simulink model "twoP"  (R2016b)
settings: Solver=FixedStepAuto  StartTime=0.0  StopTime=simstop  MaxStep=0.1  RelTol=1e-3  EnableMultiTasking=on
values from neighbouring files (symbols this model uses):
  CV01 = 100    [PIDValveTest.m]    (also in PIDtestP2m.m; loggingTest.m)
  simstop = 60*1    (= 60)    [PIDValveTest.m]    (also in PIDtestP2m.m; gatherData.m = WPtime(end)+(WPtime(end)-WPtime(end-1)))
libraries: slrtlib x5, xpcnilib x2, powerlib_meascontrol x1
settings Model: ModifiedByFormat=The MathWorks Inc.  Creator=The MathWorks, Inc.  LastModifiedBy=The MathWorks Inc.
settings SolverCC: EnableConcurrentExecution=on
settings DataIOCC: LimitDataPoints=on  SaveFormat=Array
settings OptimizationCC: BlockReduction=off  DefaultParameterBehavior=Inlined  OptimizeBlockIOStorage=off  BufferReuse=off  GlobalBufferReuse=off  ExpressionFolding=off  ExpressionDepthLimit=2147483647  LocalBlockOutputs=off  LifeSpan=inf
settings DebuggingCC: UnderspecifiedInitializationDetection=Classic  MergeDetectMultiDrivingBlocksExec=none  SolverPrmCheckMsg=warning  FcnCallInpInsideContextMsg=warning  AllowSymbolicDim=off  StateNameClashWarn=warning  SFUnexpectedBacktrackingDiag=warning  SFNoUnconditionalDefaultTransitionDiag=warning  SFExecutionAtInitializationDiag=none
settings HardwareCC: ProdBitPerPointer=32  ProdBitPerSizeT=32  ProdBitPerPtrDiffT=32  ProdLargestAtomicFloat=None  ProdWordSize=32  ProdLongLongMode=on  ProdHWDeviceType=Generic->32-bit x86 compatible
settings ModelReferenceCC: ModelReferenceNumInstancesAllowed=Single  ModelReferenceMinAlgLoopOccurrences=on  PropagateSignalLabelsOutOfModel=off
settings RTWCC: SystemTargetFile=slrt.tlc  TemplateMakefile=slrt_default_tmf  Description=Simulink Real-Time  RTWVerbose=off
settings ConfigComp: CovMetricSettings=dw  CovHtmlReporting=on  CovSaveCumulativeToWorkspaceVar=on  CovSaveSingleToWorkspaceVar=on  CovExternalEMLEnable=off  CovSFcnEnable=off

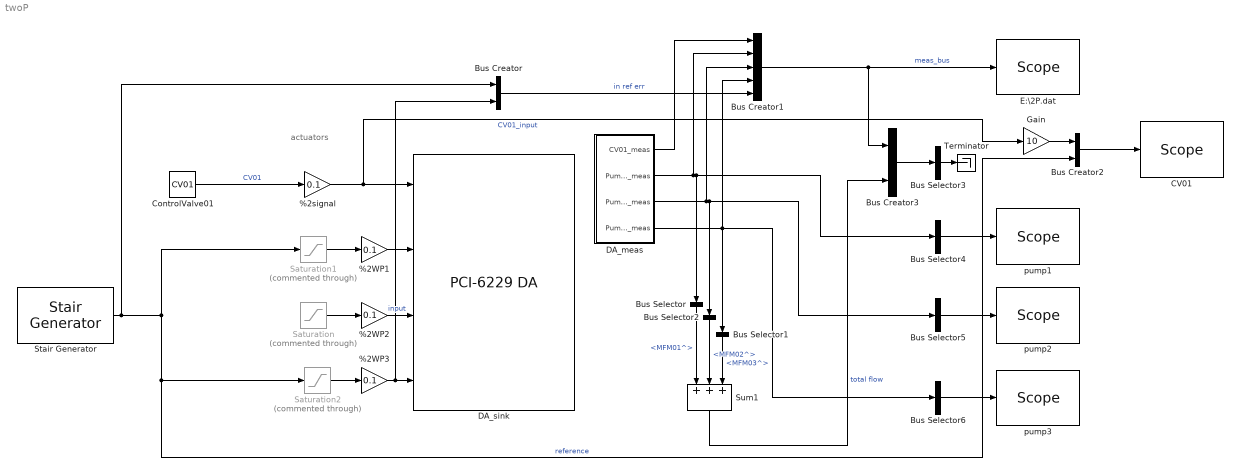
== system twoP ==
  note: actuators
  %2WP1 : Gain  Gain=0.1
  %2WP2 : Gain  Gain=0.1
  %2WP3 : Gain  Gain=0.1
  %2signal : Gain  Gain=0.1
  Bus Creator : BusCreator  Inputs=2
  Bus Creator1 : BusCreator  Inputs=5
  Bus Creator2 : BusCreator  Inputs=2
  Bus Creator3 : BusCreator  Inputs=2
  Bus Selector : BusSelector  OutputSignals=MFM01^
  Bus Selector1 : BusSelector  OutputSignals=MFM03^
  Bus Selector2 : BusSelector  OutputSignals=MFM02^
  Bus Selector3 : BusSelector  OutputSignals=meas_bus.Pump1.MFM01^  OutputAsBus=on
  Bus Selector4 : BusSelector  OutputSignals=DPT01,MFM01^  OutputAsBus=on
  Bus Selector5 : BusSelector  OutputSignals=DPT02,MFM02^  OutputAsBus=on
  Bus Selector6 : BusSelector  OutputSignals=DPT03,MFM03^  OutputAsBus=on
  CV01 : slrtlib/Displays and Logging/Scope   scopeno=4  scopetype=Target  autostart=on  viewmode=Graphical sliding  formatstr='%1.0g'  grid=on  ylimits=[0,100]  nosamples=100*simstop  noprepostsamples=0  interleave=1  triggermode=FreeRun  triggersignal=1  trigsignalfromport=on  triggerlevel=0.0  triggerslope=Either  triggerscope=1  triggersample=0  filename=E:\unused1.dat  mode=Lazy  writesize=512  autorestart=off  dynamicfilemode=off  maxwritefilesize=512*1024^2
  ControlValve01 : Constant  Value=CV01
  DA_meas : Subsystem
  DA_sink : xpcnilib/D//A/M Series/PCI-6229 DA  channel=[4 1 2 3]  reset=[1]  initValue=[0]  sampletime=0.01  slot=-1
  E:\2P.dat : slrtlib/Displays and Logging/Scope   scopeno=20  scopetype=File  autostart=on  viewmode=Graphical sliding  formatstr='%15.6f'  grid=on  ylimits=[0,0]  nosamples=100*simstop  noprepostsamples=0  interleave=1  triggermode=FreeRun  triggersignal=1  trigsignalfromport=off  triggerlevel=0.0  triggerslope=Either  triggerscope=1  triggersample=0  filename=E:\2P.dat  mode=Commit  writesize=512  autorestart=off  dynamicfilemode=off  maxwritefilesize=512*1024^2
  Gain : Gain  Gain=10
  Saturation : Saturate  Commented=through  UpperLimit=80  LowerLimit=0
  Saturation1 : Saturate  Commented=through  UpperLimit=80  LowerLimit=0
  Saturation2 : Saturate  Commented=through  UpperLimit=80  LowerLimit=0
  Stair Generator : powerlib_meascontrol/Pulse & Signal Generators/Stair Generator  t=WPtime  e=WP2  Ts=0
  Sum1 : Sum  Inputs=+++
  Terminator : Terminator
  pump1 : slrtlib/Displays and Logging/Scope   scopeno=1  scopetype=Target  autostart=on  viewmode=Graphical sliding  formatstr='%15.6f'  grid=on  ylimits=[0,0]  nosamples=100*simstop  noprepostsamples=0  interleave=1  triggermode=FreeRun  triggersignal=1  trigsignalfromport=off  triggerlevel=0.0  triggerslope=Either  triggerscope=1  triggersample=0  filename=E:\unused1.dat  mode=Lazy  writesize=512  autorestart=off  dynamicfilemode=off  maxwritefilesize=512*1024^2
  pump2 : slrtlib/Displays and Logging/Scope   scopeno=2  scopetype=Target  autostart=on  viewmode=Graphical sliding  formatstr='%15.6f'  grid=on  ylimits=[0,0]  nosamples=100*simstop  noprepostsamples=0  interleave=1  triggermode=FreeRun  triggersignal=1  trigsignalfromport=off  triggerlevel=0.0  triggerslope=Either  triggerscope=1  triggersample=0  filename=E:\unused1.dat  mode=Lazy  writesize=512  autorestart=off  dynamicfilemode=off  maxwritefilesize=512*1024^2
  pump3 : slrtlib/Displays and Logging/Scope   scopeno=3  scopetype=Target  autostart=on  viewmode=Graphical sliding  formatstr='%15.6f'  grid=on  ylimits=[0,0]  nosamples=100*simstop  noprepostsamples=0  interleave=1  triggermode=FreeRun  triggersignal=1  trigsignalfromport=off  triggerlevel=0.0  triggerslope=Either  triggerscope=1  triggersample=0  filename=E:\unused1.dat  mode=Lazy  writesize=512  autorestart=off  dynamicfilemode=off  maxwritefilesize=512*1024^2
  wires:
  %2signal/1 -> Gain/1, DA_sink/1  "CV01_input"
  %2WP1/1 -> DA_sink/2
  %2WP3/1 -> Bus Creator/2, DA_sink/4
  DA_meas/4(Pump3_meas) -> Bus Selector6/1, Bus Creator1/4, Bus Selector1/1
  DA_meas/2(Pump1_meas) -> Bus Selector4/1, Bus Selector/1, Bus Creator1/2
  DA_meas/3(Pump2_meas) -> Bus Selector5/1, Bus Selector2/1, Bus Creator1/3
  Bus Creator1/1 -> Bus Creator3/1, E:\2P.dat/1  "meas_bus"
  Bus Selector/1 -> Sum1/1  "<MFM01^>"
  Bus Selector2/1 -> Sum1/2  "<MFM02^>"
  Bus Selector1/1 -> Sum1/3  "<MFM03^>"
  Sum1/1 -> Bus Creator3/2  "total flow"
  %2WP2/1 -> DA_sink/3  "input"
  Stair Generator/1 -> Saturation1/1, Saturation2/1, Bus Creator2/2, Bus Creator/1  "reference"
  Saturation/1 -> %2WP2/1
  Bus Creator3/1 -> Bus Selector3/1
  DA_meas/1(CV01_meas) -> Bus Creator1/1
  Bus Creator/1 -> Bus Creator1/5  "in ref err"
  Saturation1/1 -> %2WP1/1
  Saturation2/1 -> %2WP3/1
  ControlValve01/1 -> %2signal/1  "CV01"
  Bus Selector4/1 -> pump1/1
  Bus Selector5/1 -> pump2/1
  Bus Selector6/1 -> pump3/1
  Bus Creator2/1 -> CV01/1
  Bus Selector3/1 -> Terminator/1
  Gain/1 -> Bus Creator2/1

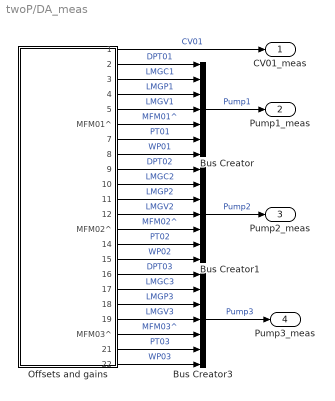
== system twoP/DA_meas ==
  Bus Creator : BusCreator  Inputs=7
  Bus Creator1 : BusCreator  Inputs=7
  Bus Creator3 : BusCreator  Inputs=7
  Offsets and gains : Subsystem
  CV01_meas : Outport
  Pump1_meas : Outport  Port=2
  Pump2_meas : Outport  Port=3
  Pump3_meas : Outport  Port=4
  wires:
  Bus Creator/1 -> Pump1_meas/1  "Pump1"
  Bus Creator1/1 -> Pump2_meas/1  "Pump2"
  Bus Creator3/1 -> Pump3_meas/1  "Pump3"
  Offsets and gains/8(8) -> Bus Creator/7  "WP01"
  Offsets and gains/9(9) -> Bus Creator1/1  "DPT02"
  Offsets and gains/4(4) -> Bus Creator/3  "LMGP1"
  Offsets and gains/2(2) -> Bus Creator/1  "DPT01"
  Offsets and gains/1(1) -> CV01_meas/1  "CV01"
  Offsets and gains/11(11) -> Bus Creator1/3  "LMGP2"
  Offsets and gains/15(15) -> Bus Creator1/7  "WP02"
  Offsets and gains/18(18) -> Bus Creator3/3  "LMGP3"
  Offsets and gains/22(22) -> Bus Creator3/7  "WP03"
  Offsets and gains/6(MFM01^) -> Bus Creator/5  "MFM01^"
  Offsets and gains/20(MFM03^) -> Bus Creator3/5  "MFM03^"
  Offsets and gains/10(10) -> Bus Creator1/2  "LMGC2"
  Offsets and gains/12(12) -> Bus Creator1/4  "LMGV2"
  Offsets and gains/13(MFM02^) -> Bus Creator1/5  "MFM02^"
  Offsets and gains/14(14) -> Bus Creator1/6  "PT02"
  Offsets and gains/19(19) -> Bus Creator3/4  "LMGV3"
  Offsets and gains/21(21) -> Bus Creator3/6  "PT03"
  Offsets and gains/16(16) -> Bus Creator3/1  "DPT03"
  Offsets and gains/17(17) -> Bus Creator3/2  "LMGC3"
  Offsets and gains/3(3) -> Bus Creator/2  "LMGC1"
  Offsets and gains/5(5) -> Bus Creator/4  "LMGV1"
  Offsets and gains/7(7) -> Bus Creator/6  "PT01"

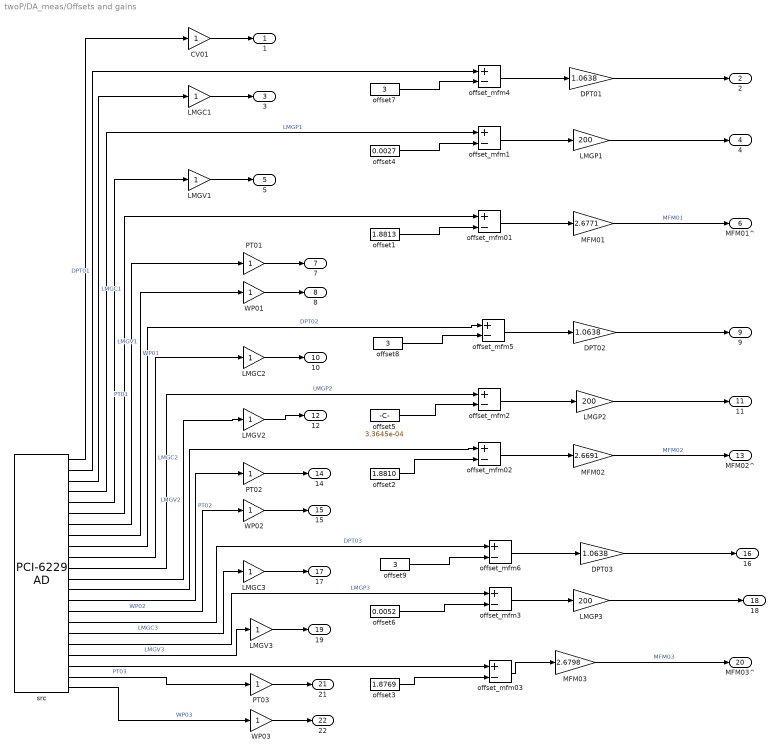
== system twoP/DA_meas/Offsets and gains ==
  CV01 : Gain
  DPT01 : Gain  Gain=1.0638
  DPT02 : Gain  Gain=1.0638
  DPT03 : Gain  Gain=1.0638
  LMGC1 : Gain
  LMGC2 : Gain
  LMGC3 : Gain
  LMGP1 : Gain  Gain=200
  LMGP2 : Gain  Gain=200
  LMGP3 : Gain  Gain=200
  LMGV1 : Gain
  LMGV2 : Gain
  LMGV3 : Gain
  MFM01 : Gain  Gain=2.6771
  MFM02 : Gain  Gain=2.6691
  MFM03 : Gain  Gain=2.6798
  PT01 : Gain
  PT02 : Gain
  PT03 : Gain
  WP01 : Gain
  WP02 : Gain
  WP03 : Gain
  offset1 : Constant  Value=1.8813
  offset2 : Constant  Value=1.8810
  offset3 : Constant  Value=1.8769
  offset4 : Constant  Value=0.0027
  offset5 : Constant  Value=3.3645e-04
  offset6 : Constant  Value=0.0052
  offset7 : Constant  Value=3
  offset8 : Constant  Value=3
  offset9 : Constant  Value=3
  offset_mfm01 : Sum  Inputs=+-
  offset_mfm02 : Sum  Inputs=+-
  offset_mfm03 : Sum  Inputs=+-
  offset_mfm{1..6} (6 alike) : Sum  Inputs=+-
  src : xpcnilib/A//D/M Series/PCI-6229 AD  channel=[4 17 5 11 8 21 24 1 18 6 12 9 22 25 2 19 7 13 10 23 26 3]  range=[10]  coupling=[0]  scantime=5e-6  sampletime=0.01  slot=-1
  1 : Outport
  2 : Outport  Port=2
  3 : Outport  Port=3
  4 : Outport  Port=4
  5 : Outport  Port=5
  MFM01^ : Outport  Port=6
  7 : Outport  Port=7
  8 : Outport  Port=8
  9 : Outport  Port=9
  10 : Outport  Port=10
  11 : Outport  Port=11
  12 : Outport  Port=12
  MFM02^ : Outport  Port=13
  14 : Outport  Port=14
  15 : Outport  Port=15
  16 : Outport  Port=16
  17 : Outport  Port=17
  18 : Outport  Port=18
  19 : Outport  Port=19
  MFM03^ : Outport  Port=20
  21 : Outport  Port=21
  22 : Outport  Port=22
  wires:
  src/18 -> offset_mfm3/1  "LMGP3"
  src/19 -> LMGV3/1  "LMGV3"
  src/22 -> WP03/1  "WP03"
  src/21 -> PT03/1  "PT03"
  src/10 -> LMGC2/1  "LMGC2"
  src/12 -> LMGV2/1  "LMGV2"
  src/15 -> WP02/1  "WP02"
  src/3 -> LMGC1/1  "LMGC1"
  src/9 -> offset_mfm5/1  "DPT02"
  src/11 -> offset_mfm2/1  "LMGP2"
  src/14 -> PT02/1  "PT02"
  src/16 -> offset_mfm6/1  "DPT03"
  src/17 -> LMGC3/1  "LMGC3"
  src/2 -> offset_mfm4/1  "DPT01"
  src/1 -> CV01/1
  MFM03/1 -> MFM03^/1  "MFM03"
  offset1/1 -> offset_mfm01/2
  src/4 -> offset_mfm1/1  "LMGP1"
  src/5 -> LMGV1/1  "LMGV1"
  src/7 -> PT01/1  "PT01"
  src/8 -> WP01/1  "WP01"
  offset3/1 -> offset_mfm03/2
  offset_mfm03/1 -> MFM03/1
  offset_mfm01/1 -> MFM01/1
  src/6 -> offset_mfm01/1
  src/20 -> offset_mfm03/1
  src/13 -> offset_mfm02/1
  offset_mfm02/1 -> MFM02/1
  offset2/1 -> offset_mfm02/2
  MFM02/1 -> MFM02^/1  "MFM02"
  MFM01/1 -> MFM01^/1  "MFM01"
  CV01/1 -> 1/1
  DPT01/1 -> 2/1
  LMGC1/1 -> 3/1
  LMGV1/1 -> 5/1
  PT01/1 -> 7/1
  WP01/1 -> 8/1
  LMGC2/1 -> 10/1
  LMGP2/1 -> 11/1
  LMGV2/1 -> 12/1
  PT02/1 -> 14/1
  WP02/1 -> 15/1
  LMGC3/1 -> 17/1
  LMGP3/1 -> 18/1
  LMGV3/1 -> 19/1
  PT03/1 -> 21/1
  WP03/1 -> 22/1
  offset4/1 -> offset_mfm1/2
  offset_mfm1/1 -> LMGP1/1
  LMGP1/1 -> 4/1
  offset_mfm2/1 -> LMGP2/1
  offset5/1 -> offset_mfm2/2
  offset_mfm3/1 -> LMGP3/1
  offset6/1 -> offset_mfm3/2
  offset7/1 -> offset_mfm4/2
  offset_mfm4/1 -> DPT01/1
  DPT02/1 -> 9/1
  offset8/1 -> offset_mfm5/2
  offset_mfm5/1 -> DPT02/1
  DPT03/1 -> 16/1
  offset9/1 -> offset_mfm6/2
  offset_mfm6/1 -> DPT03/1
